simulink model "Rohit_19EE10076_Vector"  (R2021a)
settings: Solver=ode5  StartTime=0.0  StopTime=0.1  FixedStep=2e-6  RelTol=1e-3
InitFcn:
  | Pn = 3000;
  | fg = 50;
  | 
  | Vp = 440;
  | Vs = 220;
  | rp = 100e-3;
  | Lp = 3.5e-3;
  | Rc = 1500;
  | Lm = 1500e-3;
undefined symbols (not defined in the file or in its folder): Lo_act, ro_act, Vo
libraries: spsRMSLib x28, spsVoltageMeasurementLib x16, spsCurrentMeasurementLib x12, spsLinearTransformerLib x12, spsThreePhaseProgrammableVoltageSourceLib x4, spspowerguiLib x1
settings Model: Creator=Triptendu  LastModifiedBy=hp
settings SolverCC: AlgebraicLoopSolver=TrustRegion
settings DebuggingCC: SFMachineParentedDataDiag=warning

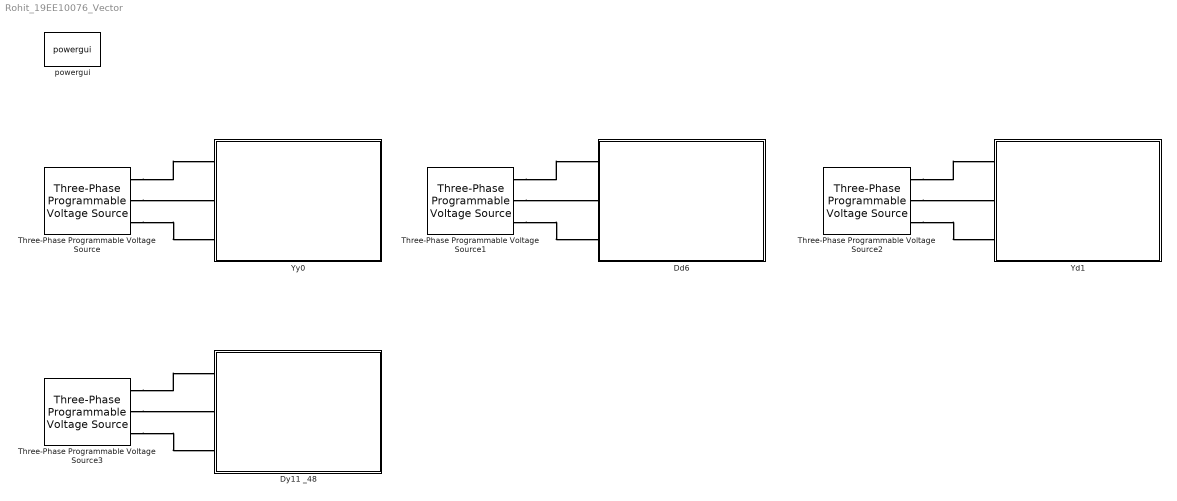
== system Rohit_19EE10076_Vector ==
  Dd6 : Subsystem
  Dy11 _48 : Subsystem
  Three-Phase Programmable Voltage Source{,1..3} (4 alike) : spsThreePhaseProgrammableVoltageSourceLib/Three-Phase Programmable Voltage Source  PositiveSequence="[440  0 50]"  VariationEntity=None  VariationType=Table of time-amplitude pairs  VariationTypeAlt=Step  VariationStep=0.5  VariationRate=10  VariationMagnitude=0.3  VariationFrequency=2  VariationTiming=[1 2]  VariationPhaseA=off  Amplitudes=[1 0.8 1.2 1.0]  TimeValues=[0 0.1 0.15 0.2]  HarmonicGeneration=off  HarmonicA=[3 0.2 -25 0]  HarmonicB=[2 0.15 35 2]  Timing="[0.05  3]"  BusType=swing  Pref=0  Qref=0  Qmin=-inf  Qmax=inf
  Yd1 : Subsystem
  Yy0 : Subsystem
  powergui : spspowerguiLib/powergui  Priority=1  SimulationMode=Discrete  SampleTime=2e-6  frequency=60  Iterations=50  frequencyindice=50  Pbase=100e6  ErrMax=1e-4  UnitsV=kV  UnitsW=MW  buscounter=0  FunctionMessages=off  echomessages=off  EnableUseOfTLC=off  CurrentSourceSwitches=off  DisableSnubberDevices=off  DisableRonSwitches=off  DisableVfSwitches=off  DisplayEquations=off  AutomaticDiscreteSolvers=off  SolverType=Backward Euler  Interpol=off  ExternalGateDelay=off  methode=off  Ts=100  x0status=blocks  SPID=on  SwTol=0  HookPort=off  NonlinearTolerance=1e-4  nMaxIteration=100  ContinueOnMaxIteration=off  RestoreLinks=warning  ResistiveCurrentMeasurement=off  Frange=[0:2:500]  Ylog=off  Xlog=on  ShowGrid=off  save=off  variable=ZData  structure=0  ZoomFFT=off  StartTime=0.0  cycles=1  DisplayStyle=1  fundamental=60  FreqAxis=off  MaxFrequency=1000  frequencyindicesteady=1  RmsSteady=1  display=off
  connections:
  Three-Phase Programmable Voltage Source/RConn1 -- Yy0/LConn1
  Three-Phase Programmable Voltage Source/RConn2 -- Yy0/LConn2
  Three-Phase Programmable Voltage Source/RConn3 -- Yy0/LConn3
  Three-Phase Programmable Voltage Source1/RConn2 -- Dd6/LConn2
  Three-Phase Programmable Voltage Source1/RConn3 -- Dd6/LConn3
  Three-Phase Programmable Voltage Source1/RConn1 -- Dd6/LConn1
  Three-Phase Programmable Voltage Source2/RConn3 -- Yd1/LConn3
  Three-Phase Programmable Voltage Source2/RConn2 -- Yd1/LConn2
  Three-Phase Programmable Voltage Source2/RConn1 -- Yd1/LConn1
  Three-Phase Programmable Voltage Source3/RConn3 -- Dy11 _48/LConn3
  Three-Phase Programmable Voltage Source3/RConn1 -- Dy11 _48/LConn1
  Three-Phase Programmable Voltage Source3/RConn2 -- Dy11 _48/LConn2

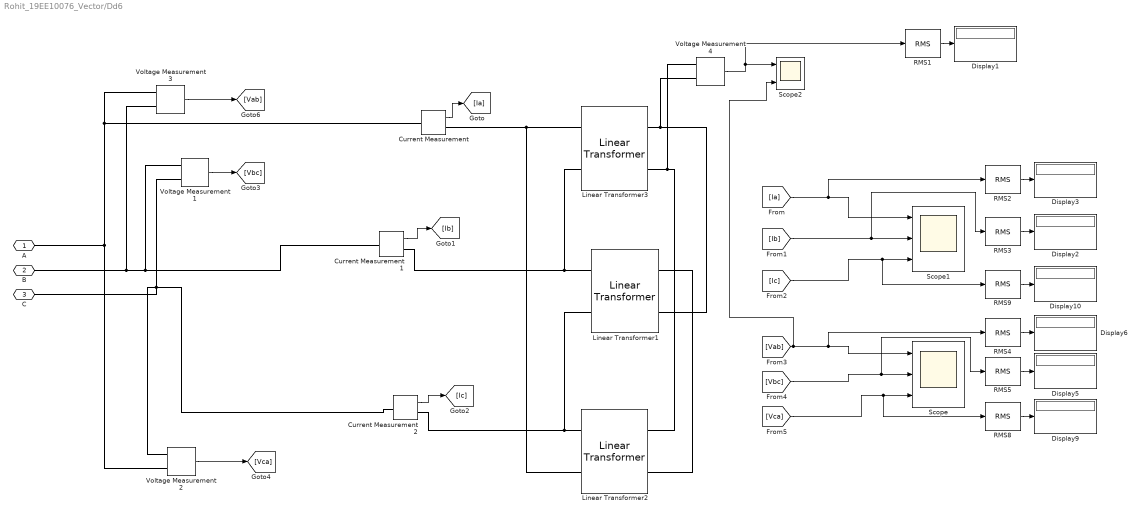
== system Rohit_19EE10076_Vector/Dd6 ==
  Current Measurement : spsCurrentMeasurementLib/Current Measurement  PhasorSimulation=off  OutputType=Complex  PSBequivalent=0
  Current Measurement1 : spsCurrentMeasurementLib/Current Measurement  PhasorSimulation=off  OutputType=Complex  PSBequivalent=0
  Current Measurement2 : spsCurrentMeasurementLib/Current Measurement  PhasorSimulation=off  OutputType=Complex  PSBequivalent=0
  Display{1..3,5..6,9..10} (7 alike) : Display
  Linear Transformer1 : spsLinearTransformerLib/Linear Transformer  UNITS=SI  NominalPower=[Pn fg]  winding1=[Vp rp Lp]  winding2=[Vs 1e-6 1e-6]  ThreeWindings=off  winding3=[Vo/2 ro_act/2 Lo_act/2]  RmLm=[Rc Lm]  Measurements=None  DataType=on
  Linear Transformer2 : spsLinearTransformerLib/Linear Transformer  UNITS=SI  NominalPower=[Pn fg]  winding1=[Vp rp Lp]  winding2=[Vs 1e-6 1e-6]  ThreeWindings=off  winding3=[Vo/2 ro_act/2 Lo_act/2]  RmLm=[Rc Lm]  Measurements=None  DataType=on
  Linear Transformer3 : spsLinearTransformerLib/Linear Transformer  UNITS=SI  NominalPower=[Pn fg]  winding1=[Vp rp Lp]  winding2=[Vs 1e-6 1e-6]  ThreeWindings=off  winding3=[Vo/2 ro_act/2 Lo_act/2]  RmLm=[Rc Lm]  Measurements=None  DataType=on
  RMS{1..5,8..9} (7 alike) : spsRMSLib/RMS  TrueRMS=on  Freq=50  RMSInit=0  Ts=0
  Scope : Scope  NumInputPorts=3
  Scope1 : Scope  NumInputPorts=3
  Scope2 : Scope  NumInputPorts=2
  Voltage Measurement{1..4} (4 alike) : spsVoltageMeasurementLib/Voltage Measurement  PhasorSimulation=off  OutputType=Complex  PSBequivalent=0
  A : PMIOPort  Side=Left
  B : PMIOPort  Port=2  Side=Left
  C : PMIOPort  Port=3  Side=Left
  wires:
  Voltage Measurement3/1 -> [Vab]
  Voltage Measurement2/1 -> [Vca]
  Voltage Measurement1/1 -> [Vbc]
  Current Measurement2/1 -> [Ic]
  Current Measurement1/1 -> [Ib]
  Current Measurement/1 -> [Ia]
  RMS9/1 -> Display10/1
  [Ia] -> RMS2/1, Scope1/1
  RMS5/1 -> Display5/1
  RMS3/1 -> Display2/1
  [Vbc] -> RMS5/1, Scope/2
  RMS4/1 -> Display6/1
  RMS2/1 -> Display3/1
  [Vca] -> RMS8/1, Scope/3
  [Ic] -> RMS9/1, Scope1/3
  [Vab] -> RMS4/1, Scope/1, Scope2/2
  RMS8/1 -> Display9/1
  [Ib] -> RMS3/1, Scope1/2
  Voltage Measurement4/1 -> RMS1/1, Scope2/1
  RMS1/1 -> Display1/1
  connections:
  Voltage Measurement1/LConn2 -- Current Measurement2/LConn1 -- Voltage Measurement2/LConn1 -- C/RConn1
  Voltage Measurement2/LConn2 -- Voltage Measurement3/LConn1 -- Current Measurement/LConn1 -- A/RConn1
  Voltage Measurement1/LConn1 -- Voltage Measurement3/LConn2 -- B/RConn1 -- Current Measurement1/LConn1
  Linear Transformer3/LConn1 -- Current Measurement/RConn1 -- Linear Transformer2/LConn2
  Linear Transformer3/LConn2 -- Current Measurement1/RConn1 -- Linear Transformer1/LConn1
  Linear Transformer2/LConn1 -- Current Measurement2/RConn1 -- Linear Transformer1/LConn2
  Linear Transformer3/RConn1 -- Voltage Measurement4/LConn2 -- Linear Transformer1/RConn2
  Linear Transformer3/RConn2 -- Voltage Measurement4/LConn1 -- Linear Transformer2/RConn1
  Linear Transformer1/RConn1 -- Linear Transformer2/RConn2

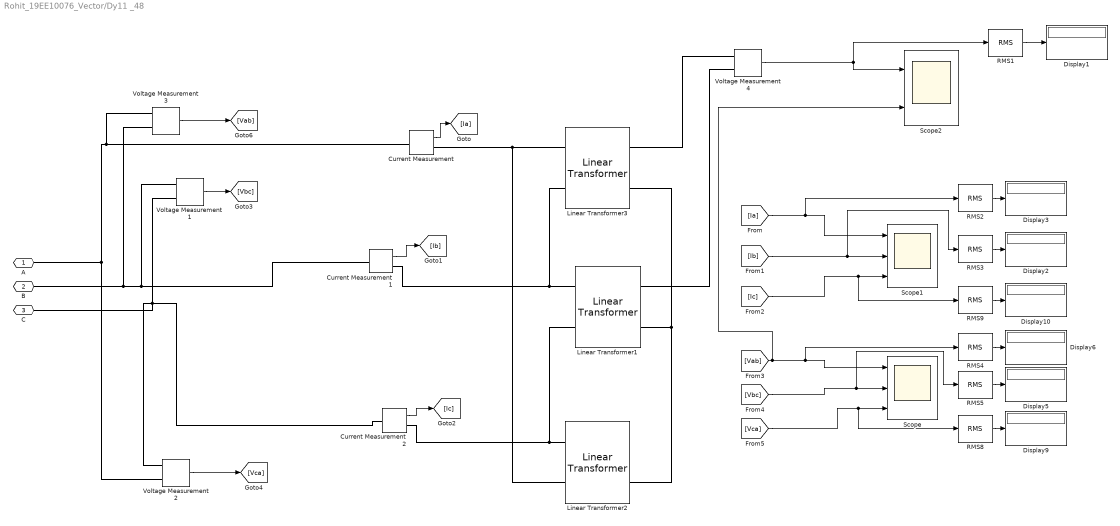
== system Rohit_19EE10076_Vector/Dy11 _48 ==
  Current Measurement : spsCurrentMeasurementLib/Current Measurement  PhasorSimulation=off  OutputType=Complex  PSBequivalent=0
  Current Measurement1 : spsCurrentMeasurementLib/Current Measurement  PhasorSimulation=off  OutputType=Complex  PSBequivalent=0
  Current Measurement2 : spsCurrentMeasurementLib/Current Measurement  PhasorSimulation=off  OutputType=Complex  PSBequivalent=0
  Display{1..3,5..6,9..10} (7 alike) : Display
  Linear Transformer1 : spsLinearTransformerLib/Linear Transformer  UNITS=SI  NominalPower=[Pn fg]  winding1=[Vp rp Lp]  winding2=[Vs 1e-6 1e-6]  ThreeWindings=off  winding3=[Vo/2 ro_act/2 Lo_act/2]  RmLm=[Rc Lm]  Measurements=None  DataType=on
  Linear Transformer2 : spsLinearTransformerLib/Linear Transformer  UNITS=SI  NominalPower=[Pn fg]  winding1=[Vp rp Lp]  winding2=[Vs 1e-6 1e-6]  ThreeWindings=off  winding3=[Vo/2 ro_act/2 Lo_act/2]  RmLm=[Rc Lm]  Measurements=None  DataType=on
  Linear Transformer3 : spsLinearTransformerLib/Linear Transformer  UNITS=SI  NominalPower=[Pn fg]  winding1=[Vp rp Lp]  winding2=[Vs 1e-6 1e-6]  ThreeWindings=off  winding3=[Vo/2 ro_act/2 Lo_act/2]  RmLm=[Rc Lm]  Measurements=None  DataType=on
  RMS{1..5,8..9} (7 alike) : spsRMSLib/RMS  TrueRMS=on  Freq=50  RMSInit=0  Ts=0
  Scope : Scope  NumInputPorts=3
  Scope1 : Scope  NumInputPorts=3
  Scope2 : Scope  NumInputPorts=2
  Voltage Measurement{1..4} (4 alike) : spsVoltageMeasurementLib/Voltage Measurement  PhasorSimulation=off  OutputType=Complex  PSBequivalent=0
  A : PMIOPort  Side=Left
  B : PMIOPort  Port=2  Side=Left
  C : PMIOPort  Port=3  Side=Left
  wires:
  Voltage Measurement3/1 -> [Vab]
  Voltage Measurement2/1 -> [Vca]
  Voltage Measurement1/1 -> [Vbc]
  Current Measurement2/1 -> [Ic]
  Current Measurement1/1 -> [Ib]
  Current Measurement/1 -> [Ia]
  RMS9/1 -> Display10/1
  [Ia] -> RMS2/1, Scope1/1
  RMS5/1 -> Display5/1
  RMS3/1 -> Display2/1
  [Vbc] -> RMS5/1, Scope/2
  RMS4/1 -> Display6/1
  RMS2/1 -> Display3/1
  [Vca] -> RMS8/1, Scope/3
  [Ic] -> RMS9/1, Scope1/3
  [Vab] -> RMS4/1, Scope/1, Scope2/2
  RMS8/1 -> Display9/1
  [Ib] -> RMS3/1, Scope1/2
  Voltage Measurement4/1 -> Scope2/1, RMS1/1
  RMS1/1 -> Display1/1
  connections:
  Voltage Measurement1/LConn2 -- Current Measurement2/LConn1 -- Voltage Measurement2/LConn1 -- C/RConn1
  Voltage Measurement2/LConn2 -- Voltage Measurement3/LConn1 -- Current Measurement/LConn1 -- A/RConn1
  Voltage Measurement1/LConn1 -- Voltage Measurement3/LConn2 -- B/RConn1 -- Current Measurement1/LConn1
  Linear Transformer3/LConn1 -- Linear Transformer2/LConn2 -- Current Measurement/RConn1
  Linear Transformer3/LConn2 -- Current Measurement1/RConn1 -- Linear Transformer1/LConn1
  Linear Transformer2/LConn1 -- Linear Transformer1/LConn2 -- Current Measurement2/RConn1
  Linear Transformer3/RConn2 -- Linear Transformer2/RConn2 -- Linear Transformer1/RConn2
  Linear Transformer3/RConn1 -- Voltage Measurement4/LConn1
  Voltage Measurement4/LConn2 -- Linear Transformer1/RConn1

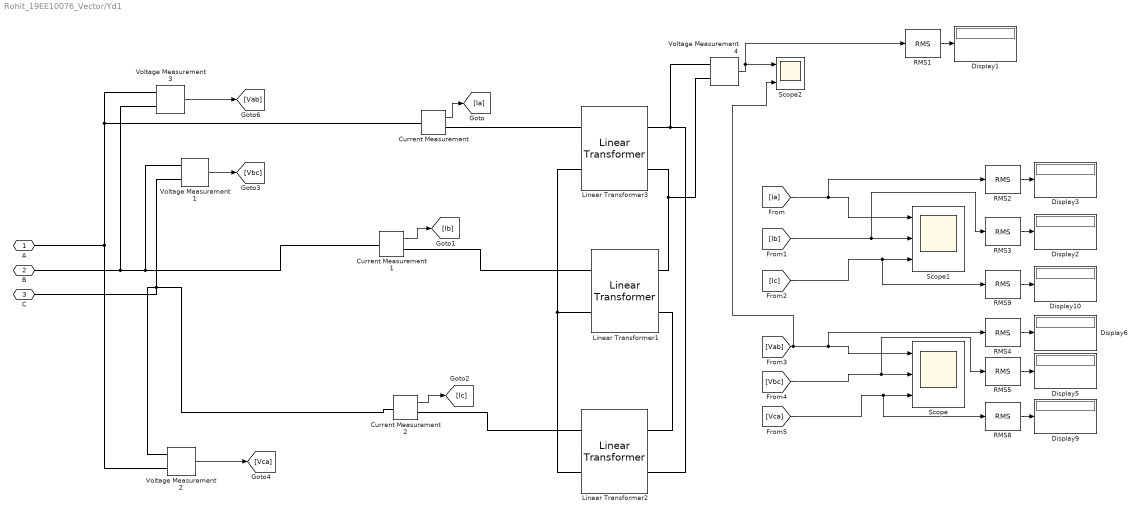
== system Rohit_19EE10076_Vector/Yd1 ==
  Current Measurement : spsCurrentMeasurementLib/Current Measurement  PhasorSimulation=off  OutputType=Complex  PSBequivalent=0
  Current Measurement1 : spsCurrentMeasurementLib/Current Measurement  PhasorSimulation=off  OutputType=Complex  PSBequivalent=0
  Current Measurement2 : spsCurrentMeasurementLib/Current Measurement  PhasorSimulation=off  OutputType=Complex  PSBequivalent=0
  Display{1..3,5..6,9..10} (7 alike) : Display
  Linear Transformer1 : spsLinearTransformerLib/Linear Transformer  UNITS=SI  NominalPower=[Pn fg]  winding1=[Vp rp Lp]  winding2=[Vs 1e-6 1e-6]  ThreeWindings=off  winding3=[Vo/2 ro_act/2 Lo_act/2]  RmLm=[Rc Lm]  Measurements=None  DataType=on
  Linear Transformer2 : spsLinearTransformerLib/Linear Transformer  UNITS=SI  NominalPower=[Pn fg]  winding1=[Vp rp Lp]  winding2=[Vs 1e-6 1e-6]  ThreeWindings=off  winding3=[Vo/2 ro_act/2 Lo_act/2]  RmLm=[Rc Lm]  Measurements=None  DataType=on
  Linear Transformer3 : spsLinearTransformerLib/Linear Transformer  UNITS=SI  NominalPower=[Pn fg]  winding1=[Vp rp Lp]  winding2=[Vs 1e-6 1e-6]  ThreeWindings=off  winding3=[Vo/2 ro_act/2 Lo_act/2]  RmLm=[Rc Lm]  Measurements=None  DataType=on
  RMS{1..5,8..9} (7 alike) : spsRMSLib/RMS  TrueRMS=on  Freq=50  RMSInit=0  Ts=0
  Scope : Scope  NumInputPorts=3
  Scope1 : Scope  NumInputPorts=3
  Scope2 : Scope  NumInputPorts=2
  Voltage Measurement{1..4} (4 alike) : spsVoltageMeasurementLib/Voltage Measurement  PhasorSimulation=off  OutputType=Complex  PSBequivalent=0
  A : PMIOPort  Side=Left
  B : PMIOPort  Port=2  Side=Left
  C : PMIOPort  Port=3  Side=Left
  wires:
  Voltage Measurement3/1 -> [Vab]
  Voltage Measurement2/1 -> [Vca]
  Voltage Measurement1/1 -> [Vbc]
  Current Measurement2/1 -> [Ic]
  Current Measurement1/1 -> [Ib]
  Current Measurement/1 -> [Ia]
  RMS9/1 -> Display10/1
  [Ia] -> RMS2/1, Scope1/1
  RMS5/1 -> Display5/1
  RMS3/1 -> Display2/1
  [Vbc] -> RMS5/1, Scope/2
  RMS4/1 -> Display6/1
  RMS2/1 -> Display3/1
  [Vca] -> RMS8/1, Scope/3
  [Ic] -> RMS9/1, Scope1/3
  [Vab] -> RMS4/1, Scope/1, Scope2/2
  RMS8/1 -> Display9/1
  [Ib] -> RMS3/1, Scope1/2
  Voltage Measurement4/1 -> RMS1/1, Scope2/1
  RMS1/1 -> Display1/1
  connections:
  Voltage Measurement1/LConn2 -- Current Measurement2/LConn1 -- Voltage Measurement2/LConn1 -- C/RConn1
  Voltage Measurement2/LConn2 -- Voltage Measurement3/LConn1 -- Current Measurement/LConn1 -- A/RConn1
  Voltage Measurement1/LConn1 -- Voltage Measurement3/LConn2 -- B/RConn1 -- Current Measurement1/LConn1
  Linear Transformer3/LConn2 -- Linear Transformer1/LConn2 -- Linear Transformer2/LConn2
  Current Measurement/RConn1 -- Linear Transformer3/LConn1
  Current Measurement1/RConn1 -- Linear Transformer1/LConn1
  Current Measurement2/RConn1 -- Linear Transformer2/LConn1
  Linear Transformer3/RConn1 -- Voltage Measurement4/LConn1 -- Linear Transformer2/RConn2
  Linear Transformer3/RConn2 -- Voltage Measurement4/LConn2 -- Linear Transformer1/RConn1
  Linear Transformer1/RConn2 -- Linear Transformer2/RConn1

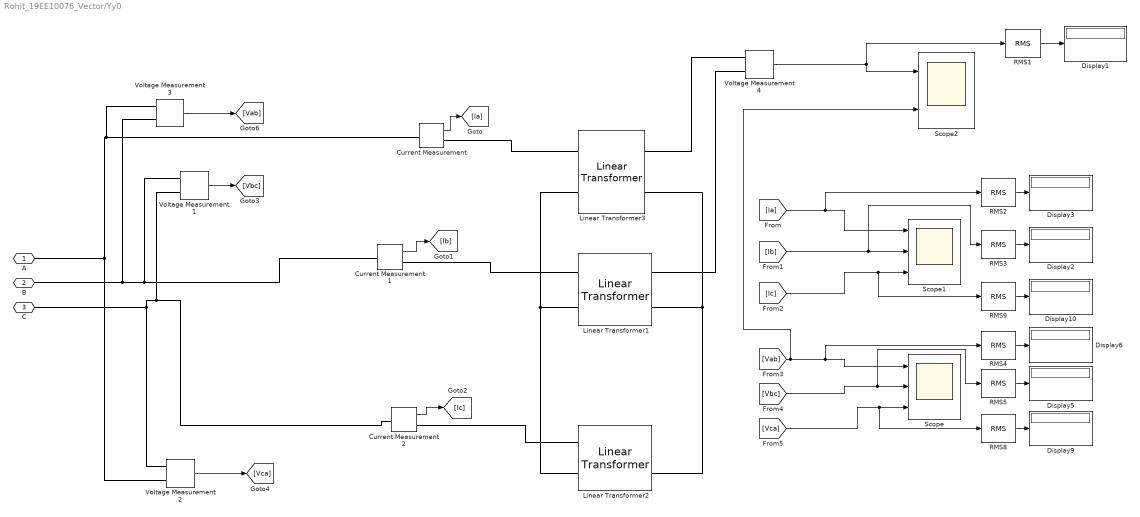
== system Rohit_19EE10076_Vector/Yy0 ==
  Current Measurement : spsCurrentMeasurementLib/Current Measurement  PhasorSimulation=off  OutputType=Complex  PSBequivalent=0
  Current Measurement1 : spsCurrentMeasurementLib/Current Measurement  PhasorSimulation=off  OutputType=Complex  PSBequivalent=0
  Current Measurement2 : spsCurrentMeasurementLib/Current Measurement  PhasorSimulation=off  OutputType=Complex  PSBequivalent=0
  Display{1..3,5..6,9..10} (7 alike) : Display
  Linear Transformer1 : spsLinearTransformerLib/Linear Transformer  UNITS=SI  NominalPower=[Pn fg]  winding1=[Vp rp Lp]  winding2=[Vs 1e-6 1e-6]  ThreeWindings=off  winding3=[Vo/2 ro_act/2 Lo_act/2]  RmLm=[Rc Lm]  Measurements=None  DataType=on
  Linear Transformer2 : spsLinearTransformerLib/Linear Transformer  UNITS=SI  NominalPower=[Pn fg]  winding1=[Vp rp Lp]  winding2=[Vs 1e-6 1e-6]  ThreeWindings=off  winding3=[Vo/2 ro_act/2 Lo_act/2]  RmLm=[Rc Lm]  Measurements=None  DataType=on
  Linear Transformer3 : spsLinearTransformerLib/Linear Transformer  UNITS=SI  NominalPower=[Pn fg]  winding1=[Vp rp Lp]  winding2=[Vs 1e-6 1e-6]  ThreeWindings=off  winding3=[Vo/2 ro_act/2 Lo_act/2]  RmLm=[Rc Lm]  Measurements=None  DataType=on
  RMS{1..5,8..9} (7 alike) : spsRMSLib/RMS  TrueRMS=on  Freq=50  RMSInit=0  Ts=0
  Scope : Scope  NumInputPorts=3
  Scope1 : Scope  NumInputPorts=3
  Scope2 : Scope  NumInputPorts=2
  Voltage Measurement{1..4} (4 alike) : spsVoltageMeasurementLib/Voltage Measurement  PhasorSimulation=off  OutputType=Complex  PSBequivalent=0
  A : PMIOPort  Side=Left
  B : PMIOPort  Port=2  Side=Left
  C : PMIOPort  Port=3  Side=Left
  wires:
  Voltage Measurement3/1 -> [Vab]
  Voltage Measurement2/1 -> [Vca]
  Voltage Measurement1/1 -> [Vbc]
  Current Measurement2/1 -> [Ic]
  Current Measurement1/1 -> [Ib]
  Current Measurement/1 -> [Ia]
  RMS9/1 -> Display10/1
  [Ia] -> RMS2/1, Scope1/1
  RMS5/1 -> Display5/1
  RMS3/1 -> Display2/1
  [Vbc] -> RMS5/1, Scope/2
  RMS4/1 -> Display6/1
  RMS2/1 -> Display3/1
  [Vca] -> RMS8/1, Scope/3
  [Ic] -> RMS9/1, Scope1/3
  RMS8/1 -> Display9/1
  [Ib] -> RMS3/1, Scope1/2
  Voltage Measurement4/1 -> Scope2/1, RMS1/1
  RMS1/1 -> Display1/1
  [Vab] -> RMS4/1, Scope/1, Scope2/2
  connections:
  Linear Transformer1/LConn2 -- Linear Transformer2/LConn2 -- Linear Transformer3/LConn2
  Current Measurement2/LConn1 -- Voltage Measurement2/LConn1 -- C/RConn1 -- Voltage Measurement1/LConn2
  Voltage Measurement2/LConn2 -- Voltage Measurement3/LConn1 -- Current Measurement/LConn1 -- A/RConn1
  Linear Transformer1/RConn2 -- Linear Transformer2/RConn2 -- Linear Transformer3/RConn2
  Current Measurement1/LConn1 -- Voltage Measurement3/LConn2 -- B/RConn1 -- Voltage Measurement1/LConn1
  Current Measurement2/RConn1 -- Linear Transformer2/LConn1
  Current Measurement/RConn1 -- Linear Transformer3/LConn1
  Current Measurement1/RConn1 -- Linear Transformer1/LConn1
  Linear Transformer1/RConn1 -- Voltage Measurement4/LConn2
  Linear Transformer3/RConn1 -- Voltage Measurement4/LConn1
